simulink model "test_mdl_NI"  (R2018a)
settings: Solver=VariableStepAuto  StartTime=0.0  StopTime=10.0  RelTol=1e-3
(part 17 of 24)

== system test_mdl_NI/CAN_Signal/ECM_DIESEL PCM PCM_HEV/EngineData_7_0x179/FuelFlw_Vl_Dsply ==
  in : Inport
  out : Outport
  wires:
  in/1 -> out/1

== system test_mdl_NI/CAN_Signal/ECM_DIESEL PCM PCM_HEV/EngineData_7_0x179/HvacAirFullOut_B_Rq ==
  in : Inport
  out : Outport
  wires:
  in/1 -> out/1

== system test_mdl_NI/CAN_Signal/ECM_DIESEL PCM PCM_HEV/EngineData_7_0x179/OdoCount ==
  in : Inport
  out : Outport
  wires:
  in/1 -> out/1

== system test_mdl_NI/CAN_Signal/ECM_DIESEL PCM PCM_HEV/EngineData_7_0x179/TrnKickDown_B_RqDrv ==
  in : Inport
  out : Outport
  wires:
  in/1 -> out/1

== system test_mdl_NI/CAN_Signal/ECM_DIESEL PCM PCM_HEV/EngineData_7_0x179/TrnManShifGear_D_IndDrv ==
  in : Inport
  out : Outport
  wires:
  in/1 -> out/1

== system test_mdl_NI/CAN_Signal/ECM_DIESEL PCM PCM_HEV/EngineData_7_0x179/TrnManShif_D_IndDrv ==
  in : Inport
  out : Outport
  wires:
  in/1 -> out/1

== system test_mdl_NI/CAN_Signal/ECM_DIESEL PCM PCM_HEV/Engine_Clutch_Data_0x42F/CluPdlPosPcMeas_D_Qf ==
  in : Inport
  out : Outport
  wires:
  in/1 -> out/1

== system test_mdl_NI/CAN_Signal/ECM_DIESEL PCM PCM_HEV/Engine_Clutch_Data_0x42F/CluPdlPos_Pc_Meas ==
  in : Inport
  out : Outport
  wires:
  in/1 -> out/1

== system test_mdl_NI/CAN_Signal/ECM_DIESEL PCM PCM_HEV/Engine_Clutch_Data_0x42F/CluPdl_PcRate_Actl ==
  in : Inport
  out : Outport
  wires:
  in/1 -> out/1

== system test_mdl_NI/CAN_Signal/ECM_DIESEL PCM PCM_HEV/Engine_Clutch_Data_0x42F/EngAoutIdl_N_Ntrl ==
  in : Inport
  out : Outport
  wires:
  in/1 -> out/1

== system test_mdl_NI/CAN_Signal/ECM_DIESEL PCM PCM_HEV/Engine_Clutch_Data_0x42F/EngAout_N_Dsply ==
  in : Inport
  out : Outport
  wires:
  in/1 -> out/1

== system test_mdl_NI/CAN_Signal/ECM_DIESEL PCM PCM_HEV/Gear_Shift_by_Wire_3/GearSelLck_D_Rq ==
  in : Inport
  out : Outport
  wires:
  in/1 -> out/1

== system test_mdl_NI/CAN_Signal/ECM_DIESEL PCM PCM_HEV/Gear_Shift_by_Wire_3/PrkBrkActv_D_RqTrnGear ==
  in : Inport
  out : Outport
  wires:
  in/1 -> out/1

== system test_mdl_NI/CAN_Signal/ECM_DIESEL PCM PCM_HEV/Gear_Shift_by_Wire_3/TrnCmdCnt_B_Actl ==
  in : Inport
  out : Outport
  wires:
  in/1 -> out/1

== system test_mdl_NI/CAN_Signal/ECM_DIESEL PCM PCM_HEV/Gear_Shift_by_Wire_3/TrnCmdState_B_Actl ==
  in : Inport
  out : Outport
  wires:
  in/1 -> out/1

== system test_mdl_NI/CAN_Signal/ECM_DIESEL PCM PCM_HEV/Gear_Shift_by_Wire_3/TrnDtpCmd_D_Actl ==
  in : Inport
  out : Outport
  wires:
  in/1 -> out/1

== system test_mdl_NI/CAN_Signal/ECM_DIESEL PCM PCM_HEV/Gear_Shift_by_Wire_3/TrnGearCmd_No_Cnt ==
  in : Inport
  out : Outport
  wires:
  in/1 -> out/1

== system test_mdl_NI/CAN_Signal/ECM_DIESEL PCM PCM_HEV/Gear_Shift_by_Wire_3/TrnGearCmd_No_Cs ==
  in : Inport
  out : Outport
  wires:
  in/1 -> out/1

== system test_mdl_NI/CAN_Signal/ECM_DIESEL PCM PCM_HEV/Gear_Shift_by_Wire_3/TrnGearCmd_Pc_ActlPt ==
  in : Inport
  out : Outport
  wires:
  in/1 -> out/1

== system test_mdl_NI/CAN_Signal/ECM_DIESEL PCM PCM_HEV/Gear_Shift_by_Wire_3/TrnGearMsgTxt_D_Rq ==
  in : Inport
  out : Outport
  wires:
  in/1 -> out/1

== system test_mdl_NI/CAN_Signal/ECM_DIESEL PCM PCM_HEV/Gear_Shift_by_Wire_3/TrnGearNtmAllow_B_Stat ==
  in : Inport
  out : Outport
  wires:
  in/1 -> out/1

== system test_mdl_NI/CAN_Signal/ECM_DIESEL PCM PCM_HEV/Gear_Shift_by_Wire_3/TrnGear_D_RqPt ==
  in : Inport
  out : Outport
  wires:
  in/1 -> out/1

== system test_mdl_NI/CAN_Signal/ECM_DIESEL PCM PCM_HEV/Gear_Shift_by_Wire_3/TrnLvrV_D_Rq ==
  in : Inport
  out : Outport
  wires:
  in/1 -> out/1

== system test_mdl_NI/CAN_Signal/ECM_DIESEL PCM PCM_HEV/Gear_Shift_by_Wire_3/TrnNtrlTowCmd_D_Actl ==
  in : Inport
  out : Outport
  wires:
  in/1 -> out/1

== system test_mdl_NI/CAN_Signal/ECM_DIESEL PCM PCM_HEV/Gear_Shift_by_Wire_3/TrnSbwSysHlth_D_Actl ==
  in : Inport
  out : Outport
  wires:
  in/1 -> out/1

== system test_mdl_NI/CAN_Signal/ECM_DIESEL PCM PCM_HEV/Gear_Shift_by_Wire_3/TrnValidGear_D_Cnfm ==
  in : Inport
  out : Outport
  wires:
  in/1 -> out/1

== system test_mdl_NI/CAN_Signal/ECM_DIESEL PCM PCM_HEV/Global_PATS_TargetInfo_0x47/immoTarget1Cmd ==
  in : Inport
  out : Outport
  wires:
  in/1 -> out/1

== system test_mdl_NI/CAN_Signal/ECM_DIESEL PCM PCM_HEV/Global_PATS_TargetInfo_0x47/immoTarget1Data ==
  in : Inport
  out : Outport
  wires:
  in/1 -> out/1

== system test_mdl_NI/CAN_Signal/ECM_DIESEL PCM PCM_HEV/Global_PATS_TargetInfo_0x47/immoTarget1Status ==
  in : Inport
  out : Outport
  wires:
  in/1 -> out/1

== system test_mdl_NI/CAN_Signal/ECM_DIESEL PCM PCM_HEV/HEV_Powertrain_Data2/BattTracCnnct_D_Rq ==
  in : Inport
  out : Outport
  wires:
  in/1 -> out/1

== system test_mdl_NI/CAN_Signal/ECM_DIESEL PCM PCM_HEV/HEV_Powertrain_Data2/PrplTqMnRgen_B_Actl ==
  in : Inport
  out : Outport
  wires:
  in/1 -> out/1

== system test_mdl_NI/CAN_Signal/ECM_DIESEL PCM PCM_HEV/HEV_Powertrain_Data2/WhlDirAvgDrv_D_Actl ==
  in : Inport
  out : Outport
  wires:
  in/1 -> out/1

== system test_mdl_NI/CAN_Signal/ECM_DIESEL PCM PCM_HEV/PCM_AutoSar_NetworkMgmt_0x595/PCM_AutoSarNMControl ==
  in : Inport
  out : Outport
  wires:
  in/1 -> out/1

== system test_mdl_NI/CAN_Signal/ECM_DIESEL PCM PCM_HEV/PCM_AutoSar_NetworkMgmt_0x595/PCM_AutoSarNMNodeId ==
  in : Inport
  out : Outport
  wires:
  in/1 -> out/1

== system test_mdl_NI/CAN_Signal/ECM_DIESEL PCM PCM_HEV/PCM_AutoSar_NetworkMgmt_0x595/PCM_AutoSarNMReserved1 ==
  in : Inport
  out : Outport
  wires:
  in/1 -> out/1

== system test_mdl_NI/CAN_Signal/ECM_DIESEL PCM PCM_HEV/PCM_AutoSar_NetworkMgmt_0x595/PCM_AutoSarNMReserved2 ==
  in : Inport
  out : Outport
  wires:
  in/1 -> out/1

== system test_mdl_NI/CAN_Signal/ECM_DIESEL PCM PCM_HEV/PCM_AutoSar_NetworkMgmt_0x595/PCM_AutoSarNMReserved3 ==
  in : Inport
  out : Outport
  wires:
  in/1 -> out/1

== system test_mdl_NI/CAN_Signal/ECM_DIESEL PCM PCM_HEV/PCM_AutoSar_NetworkMgmt_0x595/PCM_AutoSarNMReserved4 ==
  in : Inport
  out : Outport
  wires:
  in/1 -> out/1

== system test_mdl_NI/CAN_Signal/ECM_DIESEL PCM PCM_HEV/PCM_AutoSar_NetworkMgmt_0x595/PCM_GWNMProxy ==
  in : Inport
  out : Outport
  wires:
  in/1 -> out/1

== system test_mdl_NI/CAN_Signal/ECM_DIESEL PCM PCM_HEV/PCM_AutoSar_NetworkMgmt_0x595/PCM_GWOnBoardTester ==
  in : Inport
  out : Outport
  wires:
  in/1 -> out/1

== system test_mdl_NI/CAN_Signal/ECM_DIESEL PCM PCM_HEV/PCM_Rapid_Data_Response_1_0x6A0/UUDTPCMResponse1 ==
  in : Inport
  out : Outport
  wires:
  in/1 -> out/1

== system test_mdl_NI/CAN_Signal/ECM_DIESEL PCM PCM_HEV/PowertrainData_10/GearEngag_D_Actl ==
  in : Inport
  out : Outport
  wires:
  in/1 -> out/1

== system test_mdl_NI/CAN_Signal/ECM_DIESEL PCM PCM_HEV/PowertrainData_10/GearLvr_D_ActlDrv ==
  in : Inport
  out : Outport
  wires:
  in/1 -> out/1

== system test_mdl_NI/CAN_Signal/ECM_DIESEL PCM PCM_HEV/PowertrainData_10/GearPos_D_Actl ==
  in : Inport
  out : Outport
  wires:
  in/1 -> out/1

== system test_mdl_NI/CAN_Signal/ECM_DIESEL PCM PCM_HEV/PowertrainData_10/GearPos_D_Trg ==
  in : Inport
  out : Outport
  wires:
  in/1 -> out/1

== system test_mdl_NI/CAN_Signal/ECM_DIESEL PCM PCM_HEV/PowertrainData_10/GearPos_No_Cnt ==
  in : Inport
  out : Outport
  wires:
  in/1 -> out/1

== system test_mdl_NI/CAN_Signal/ECM_DIESEL PCM PCM_HEV/PowertrainData_10/GearPos_No_Cs ==
  in : Inport
  out : Outport
  wires:
  in/1 -> out/1

== system test_mdl_NI/CAN_Signal/ECM_DIESEL PCM PCM_HEV/PowertrainData_10/TrnIgnOffDly_T_Rq ==
  in : Inport
  out : Outport
  wires:
  in/1 -> out/1

== system test_mdl_NI/CAN_Signal/ECM_DIESEL PCM PCM_HEV/PowertrainData_10/TrnPrkSys_D_Actl ==
  in : Inport
  out : Outport
  wires:
  in/1 -> out/1

== system test_mdl_NI/CAN_Signal/ECM_DIESEL PCM PCM_HEV/PowertrainData_10/TrnRng_D_Rq ==
  in : Inport
  out : Outport
  wires:
  in/1 -> out/1

== system test_mdl_NI/CAN_Signal/ECM_DIESEL PCM PCM_HEV/PowertrainData_1_0x421/AirCondFluidHi_P_Actl ==
  in : Inport
  out : Outport
  wires:
  in/1 -> out/1

== system test_mdl_NI/CAN_Signal/ECM_DIESEL PCM PCM_HEV/PowertrainData_1_0x421/CoolantFanStepAct ==
  in : Inport
  out : Outport
  wires:
  in/1 -> out/1

== system test_mdl_NI/CAN_Signal/ECM_DIESEL PCM PCM_HEV/PowertrainData_1_0x421/ECMMILRequest ==
  in : Inport
  out : Outport
  wires:
  in/1 -> out/1

== system test_mdl_NI/CAN_Signal/ECM_DIESEL PCM PCM_HEV/PowertrainData_1_0x421/EngIdlShutDown_D_Stat ==
  in : Inport
  out : Outport
  wires:
  in/1 -> out/1

== system test_mdl_NI/CAN_Signal/ECM_DIESEL PCM PCM_HEV/PowertrainData_1_0x421/EngIdlShutDwnTxt_D_Rq ==
  in : Inport
  out : Outport
  wires:
  in/1 -> out/1

== system test_mdl_NI/CAN_Signal/ECM_DIESEL PCM PCM_HEV/PowertrainData_1_0x421/FUEL_ALCOHOL_PERCNT ==
  in : Inport
  out : Outport
  wires:
  in/1 -> out/1

== system test_mdl_NI/CAN_Signal/ECM_DIESEL PCM PCM_HEV/PowertrainData_1_0x421/FohEng_D_Rq ==
  in : Inport
  out : Outport
  wires:
  in/1 -> out/1

== system test_mdl_NI/CAN_Signal/ECM_DIESEL PCM PCM_HEV/PowertrainData_1_0x421/OilPressureWarning ==
  in : Inport
  out : Outport
  wires:
  in/1 -> out/1

== system test_mdl_NI/CAN_Signal/ECM_DIESEL PCM PCM_HEV/PowertrainData_1_0x421/TrnTotLss_Tq_Est ==
  in : Inport
  out : Outport
  wires:
  in/1 -> out/1

== system test_mdl_NI/CAN_Signal/ECM_DIESEL PCM PCM_HEV/PowertrainData_1_0x421/TrnTotTq_Rt_Est ==
  in : Inport
  out : Outport
  wires:
  in/1 -> out/1

== system test_mdl_NI/CAN_Signal/ECM_DIESEL PCM PCM_HEV/PowertrainData_1_0x421/VehVLimActv_B_Actl ==
  in : Inport
  out : Outport
  wires:
  in/1 -> out/1

== system test_mdl_NI/CAN_Signal/ECM_DIESEL PCM PCM_HEV/PowertrainData_1_0x421/VehVLimStat_D_Actl ==
  in : Inport
  out : Outport
  wires:
  in/1 -> out/1

== system test_mdl_NI/CAN_Signal/ECM_DIESEL PCM PCM_HEV/PowertrainData_2_0x42D/ApedPos_Pc_ActlDiag ==
  in : Inport
  out : Outport
  wires:
  in/1 -> out/1

== system test_mdl_NI/CAN_Signal/ECM_DIESEL PCM PCM_HEV/PowertrainData_2_0x42D/EngAirIn_Te_Actl ==
  in : Inport
  out : Outport
  wires:
  in/1 -> out/1

== system test_mdl_NI/CAN_Signal/ECM_DIESEL PCM PCM_HEV/PowertrainData_2_0x42D/EngClnt_Te_ActlDiag ==
  in : Inport
  out : Outport
  wires:
  in/1 -> out/1

== system test_mdl_NI/CAN_Signal/ECM_DIESEL PCM PCM_HEV/PowertrainData_2_0x42D/EngLoad_Pc_CalcDiag ==
  in : Inport
  out : Outport
  wires:
  in/1 -> out/1

== system test_mdl_NI/CAN_Signal/ECM_DIESEL PCM PCM_HEV/PowertrainData_2_0x42D/EngMsgTxt_D_Rq ==
  in : Inport
  out : Outport
  wires:
  in/1 -> out/1

== system test_mdl_NI/CAN_Signal/ECM_DIESEL PCM PCM_HEV/PowertrainData_2_0x42D/GrllShtrPos_B_Falt ==
  in : Inport
  out : Outport
  wires:
  in/1 -> out/1

== system test_mdl_NI/CAN_Signal/ECM_DIESEL PCM PCM_HEV/PowertrainData_2_0x42D/GrllShtrPos_D_Cmd ==
  in : Inport
  out : Outport
  wires:
  in/1 -> out/1

== system test_mdl_NI/CAN_Signal/ECM_DIESEL PCM PCM_HEV/PowertrainData_2_0x42D/IsaOffst_D_Stat ==
  in : Inport
  out : Outport
  wires:
  in/1 -> out/1

== system test_mdl_NI/CAN_Signal/ECM_DIESEL PCM PCM_HEV/PowertrainData_2_0x42D/ObdWarmUp_B_Complt ==
  in : Inport
  out : Outport
  wires:
  in/1 -> out/1

== system test_mdl_NI/CAN_Signal/ECM_DIESEL PCM PCM_HEV/PowertrainData_2_0x42D/SlMde_D_RqDsply ==
  in : Inport
  out : Outport
  wires:
  in/1 -> out/1

== system test_mdl_NI/CAN_Signal/ECM_DIESEL PCM PCM_HEV/PowertrainData_2_0x42D/SlMde_D_Stat ==
  in : Inport
  out : Outport
  wires:
  in/1 -> out/1

== system test_mdl_NI/CAN_Signal/ECM_DIESEL PCM PCM_HEV/PowertrainData_3_0x43E/BattULoChrg_U_Cmd ==
  in : Inport
  out : Outport
  wires:
  in/1 -> out/1

== system test_mdl_NI/CAN_Signal/ECM_DIESEL PCM PCM_HEV/PowertrainData_3_0x43E/ElLoadCtl_D_Rq ==
  in : Inport
  out : Outport
  wires:
  in/1 -> out/1

== system test_mdl_NI/CAN_Signal/ECM_DIESEL PCM PCM_HEV/PowertrainData_3_0x43E/EngMnfld_P_Actl ==
  in : Inport
  out : Outport
  wires:
  in/1 -> out/1

== system test_mdl_NI/CAN_Signal/ECM_DIESEL PCM PCM_HEV/PowertrainData_3_0x43E/FuelPumpPwr_B_Rq ==
  in : Inport
  out : Outport
  wires:
  in/1 -> out/1

== system test_mdl_NI/CAN_Signal/ECM_DIESEL PCM PCM_HEV/PowertrainData_6_0x205/BrkTot_Tq_RqFapLc ==
  in : Inport
  out : Outport
  wires:
  in/1 -> out/1

== system test_mdl_NI/CAN_Signal/ECM_DIESEL PCM PCM_HEV/PowertrainData_6_0x205/FapLc_B_Err ==
  in : Inport
  out : Outport
  wires:
  in/1 -> out/1

== system test_mdl_NI/CAN_Signal/ECM_DIESEL PCM PCM_HEV/PowertrainData_6_0x205/TrnAin_Pc_RqDrv ==
  in : Inport
  out : Outport
  wires:
  in/1 -> out/1

== system test_mdl_NI/CAN_Signal/ECM_DIESEL PCM PCM_HEV/PowertrainData_7_0x41F/EcoCochA_Pc_Dsply ==
  in : Inport
  out : Outport
  wires:
  in/1 -> out/1

== system test_mdl_NI/CAN_Signal/ECM_DIESEL PCM PCM_HEV/PowertrainData_7_0x41F/EcoCochCrus_Pc_Dsply ==
  in : Inport
  out : Outport
  wires:
  in/1 -> out/1

== system test_mdl_NI/CAN_Signal/ECM_DIESEL PCM PCM_HEV/PowertrainData_7_0x41F/EcoCochDecel_Pc_Dsply ==
  in : Inport
  out : Outport
  wires:
  in/1 -> out/1

== system test_mdl_NI/CAN_Signal/ECM_DIESEL PCM PCM_HEV/PowertrainData_7_0x41F/EcoCochIdlFuel_Pc_Dsply ==
  in : Inport
  out : Outport
  wires:
  in/1 -> out/1

== system test_mdl_NI/CAN_Signal/ECM_DIESEL PCM PCM_HEV/PowertrainData_7_0x41F/EcoCochInstNeg_B_Dsply ==
  in : Inport
  out : Outport
  wires:
  in/1 -> out/1

== system test_mdl_NI/CAN_Signal/ECM_DIESEL PCM PCM_HEV/PowertrainData_7_0x41F/EcoCochInst_Pc_Dsply ==
  in : Inport
  out : Outport
  wires:
  in/1 -> out/1

== system test_mdl_NI/CAN_Signal/ECM_DIESEL PCM PCM_HEV/PowertrainData_7_0x41F/EcoCochShif_Pc_Dsply ==
  in : Inport
  out : Outport
  wires:
  in/1 -> out/1

== system test_mdl_NI/CAN_Signal/ECM_DIESEL PCM PCM_HEV/PowertrainData_9_0x44C/AutoTowActv_B_Stat ==
  in : Inport
  out : Outport
  wires:
  in/1 -> out/1

== system test_mdl_NI/CAN_Signal/ECM_DIESEL PCM PCM_HEV/PowertrainData_9_0x44C/AutoTowAllw_D_StatMnu ==
  in : Inport
  out : Outport
  wires:
  in/1 -> out/1

== system test_mdl_NI/CAN_Signal/ECM_DIESEL PCM PCM_HEV/PowertrainData_9_0x44C/GrossTrainWeight_M_Est ==
  in : Inport
  out : Outport
  wires:
  in/1 -> out/1

== system test_mdl_NI/CAN_Signal/ECM_DIESEL PCM PCM_HEV/PowertrainData_9_0x44C/TrailCtlPt_B_Falt ==
  in : Inport
  out : Outport
  wires:
  in/1 -> out/1

== system test_mdl_NI/CAN_Signal/ECM_DIESEL PCM PCM_HEV/PowertrainData_9_0x44C/Veh_V_DsplyTrailCtlSet ==
  in : Inport
  out : Outport
  wires:
  in/1 -> out/1

== system test_mdl_NI/CAN_Signal/ECM_DIESEL PCM PCM_HEV/PowertrainData_9_0x44C/WakeAlarm1_B_Typ ==
  in : Inport
  out : Outport
  wires:
  in/1 -> out/1

== system test_mdl_NI/CAN_Signal/ECM_DIESEL PCM PCM_HEV/PowertrainData_9_0x44C/WakeAlarm1_T_Rq ==
  in : Inport
  out : Outport
  wires:
  in/1 -> out/1

== system test_mdl_NI/CAN_Signal/ECM_DIESEL PCM PCM_HEV/Powertrain_Data_4_0x424/BpedDrvMsgTxt_B_Dsply ==
  in : Inport
  out : Outport
  wires:
  in/1 -> out/1

== system test_mdl_NI/CAN_Signal/ECM_DIESEL PCM PCM_HEV/Powertrain_Data_4_0x424/FuelLvlWarn_D_ActlEng ==
  in : Inport
  out : Outport
  wires:
  in/1 -> out/1

== system test_mdl_NI/CAN_Signal/ECM_DIESEL PCM PCM_HEV/Powertrain_Data_4_0x424/FuelLvl_Pc_DsplyEng ==
  in : Inport
  out : Outport
  wires:
  in/1 -> out/1

== system test_mdl_NI/CAN_Signal/ECM_DIESEL PCM PCM_HEV/Powertrain_Data_4_0x424/FuelRange_L_DsplyEng ==
  in : Inport
  out : Outport
  wires:
  in/1 -> out/1

== system test_mdl_NI/CAN_Signal/ECM_DIESEL PCM PCM_HEV/Powertrain_Data_4_0x424/RearDiffOilTeWarn_B_Rq ==
  in : Inport
  out : Outport
  wires:
  in/1 -> out/1

== system test_mdl_NI/CAN_Signal/ECM_DIESEL PCM PCM_HEV/Powertrain_Data_4_0x424/RearDiffOil_Te_Actl ==
  in : Inport
  out : Outport
  wires:
  in/1 -> out/1

== system test_mdl_NI/CAN_Signal/ECM_DIESEL PCM PCM_HEV/Powertrain_Data_4_0x424/SelDrvMdePt_D_Stat ==
  in : Inport
  out : Outport
  wires:
  in/1 -> out/1

== system test_mdl_NI/CAN_Signal/ECM_DIESEL PCM PCM_HEV/Powertrain_Data_5_0x43F/FapLcActv_B_Stat ==
  in : Inport
  out : Outport
  wires:
  in/1 -> out/1

== system test_mdl_NI/CAN_Signal/ECM_DIESEL PCM PCM_HEV/Powertrain_Data_5_0x43F/FapLcInhbt_B_Rq ==
  in : Inport
  out : Outport
  wires:
  in/1 -> out/1

== system test_mdl_NI/CAN_Signal/ECM_DIESEL PCM PCM_HEV/Powertrain_Data_5_0x43F/FapLcMaxGrdAbrt_B_Stat ==
  in : Inport
  out : Outport
  wires:
  in/1 -> out/1

== system test_mdl_NI/CAN_Signal/ECM_DIESEL PCM PCM_HEV/Powertrain_Data_5_0x43F/FapLcMaxGrdInhbt_B_Stat ==
  in : Inport
  out : Outport
  wires:
  in/1 -> out/1

== system test_mdl_NI/CAN_Signal/ECM_DIESEL PCM PCM_HEV/Powertrain_Data_5_0x43F/FapLcObstcl_B_Stat ==
  in : Inport
  out : Outport
  wires:
  in/1 -> out/1

== system test_mdl_NI/CAN_Signal/ECM_DIESEL PCM PCM_HEV/Powertrain_Data_5_0x43F/FapLcPrchgBrk_B_Rq ==
  in : Inport
  out : Outport
  wires:
  in/1 -> out/1

== system test_mdl_NI/CAN_Signal/ECM_DIESEL PCM PCM_HEV/Powertrain_Data_5_0x43F/FapLcStopHold_B_Rq ==
  in : Inport
  out : Outport
  wires:
  in/1 -> out/1

== system test_mdl_NI/CAN_Signal/ECM_DIESEL PCM PCM_HEV/Stop_Start_0x166/AutoStopPtDelta_I_Est ==
  in : Inport
  out : Outport
  wires:
  in/1 -> out/1

== system test_mdl_NI/CAN_Signal/ECM_DIESEL PCM PCM_HEV/Stop_Start_0x166/HiElPwInhbt_B_Stat ==
  in : Inport
  out : Outport
  wires:
  in/1 -> out/1

== system test_mdl_NI/CAN_Signal/ECM_DIESEL PCM PCM_HEV/Stop_Start_0x166/OdoTripVerify_L_Actl ==
  in : Inport
  out : Outport
  wires:
  in/1 -> out/1

== system test_mdl_NI/CAN_Signal/ECM_DIESEL PCM PCM_HEV/Stop_Start_0x166/StopStrtDrvMde_D_Indic ==
  in : Inport
  out : Outport
  wires:
  in/1 -> out/1

== system test_mdl_NI/CAN_Signal/ECM_DIESEL PCM PCM_HEV/Stop_Start_0x166/StopStrtIODTxt_D_Rq ==
  in : Inport
  out : Outport
  wires:
  in/1 -> out/1

== system test_mdl_NI/CAN_Signal/ECM_DIESEL PCM PCM_HEV/Stop_Start_0x166/StopStrtMsgTxt_D_Rq ==
  in : Inport
  out : Outport
  wires:
  in/1 -> out/1

== system test_mdl_NI/CAN_Signal/ECM_DIESEL PCM PCM_HEV/Stop_Start_0x166/StopStrtStdby_D_Indic ==
  in : Inport
  out : Outport
  wires:
  in/1 -> out/1

== system test_mdl_NI/CAN_Signal/ECM_DIESEL PCM PCM_HEV/TesterPhysicalResPCM_0x7E8/TesterPhysicalResPCM ==
  in : Inport
  out : Outport
  wires:
  in/1 -> out/1

== system test_mdl_NI/CAN_Signal/ECM_DIESEL PCM PCM_HEV/TorqueDataEngFlags_0x200/PrplWhlTotTqRq_No_Cnt ==
  in : Inport
  out : Outport
  wires:
  in/1 -> out/1

== system test_mdl_NI/CAN_Signal/ECM_DIESEL PCM PCM_HEV/TorqueDataEngFlags_0x200/PrplWhlTotTqRq_No_Cs ==
  in : Inport
  out : Outport
  wires:
  in/1 -> out/1

== system test_mdl_NI/CAN_Signal/ECM_DIESEL PCM PCM_HEV/TorqueDataEngFlags_0x200/PrplWhlTot_Tq_LimMn ==
  in : Inport
  out : Outport
  wires:
  in/1 -> out/1

== system test_mdl_NI/CAN_Signal/ECM_DIESEL PCM PCM_HEV/TorqueDataEngFlags_0x200/PrplWhlTot_Tq_Rq ==
  in : Inport
  out : Outport
  wires:
  in/1 -> out/1

== system test_mdl_NI/CAN_Signal/ECM_DIESEL PCM PCM_HEV/TorqueDataEngFlags_0x200/PtDrvMde_D_Stat ==
  in : Inport
  out : Outport
  wires:
  in/1 -> out/1

== system test_mdl_NI/CAN_Signal/ECM_DIESEL PCM PCM_HEV/TransGearData/GboxOil_Te_Actl ==
  in : Inport
  out : Outport
  wires:
  in/1 -> out/1

== system test_mdl_NI/CAN_Signal/ECM_DIESEL PCM PCM_HEV/TransGearData/GearLvrPos_D_Actl ==
  in : Inport
  out : Outport
  wires:
  in/1 -> out/1

== system test_mdl_NI/CAN_Signal/ECM_DIESEL PCM PCM_HEV/TransGearData/SelDrvMdeSwtch_D_Stat3 ==
  in : Inport
  out : Outport
  wires:
  in/1 -> out/1

== system test_mdl_NI/CAN_Signal/ECM_DIESEL PCM PCM_HEV/TransGearData/TrnShifActv_B_Actl ==
  in : Inport
  out : Outport
  wires:
  in/1 -> out/1

== system test_mdl_NI/CAN_Signal/ECM_DIESEL PCM PCM_HEV/TransGearData/TrnSrvcRqd_B_Rq ==
  in : Inport
  out : Outport
  wires:
  in/1 -> out/1

== system test_mdl_NI/CAN_Signal/ECM_DIESEL PCM PCM_HEV/VehicleOperatingModes_0x167/ElPw_D_Stat ==
  in : Inport
  out : Outport
  wires:
  in/1 -> out/1

== system test_mdl_NI/CAN_Signal/ECM_DIESEL PCM PCM_HEV/VehicleOperatingModes_0x167/ElPw_D_StatStrtStop ==
  in : Inport
  out : Outport
  wires:
  in/1 -> out/1

== system test_mdl_NI/CAN_Signal/ECM_DIESEL PCM PCM_HEV/VehicleOperatingModes_0x167/Eng_D_Stat ==
  in : Inport
  out : Outport
  wires:
  in/1 -> out/1

== system test_mdl_NI/CAN_Signal/ECM_DIESEL PCM PCM_HEV/VehicleOperatingModes_0x167/PlgActvArb_B_Actl ==
  in : Inport
  out : Outport
  wires:
  in/1 -> out/1

== system test_mdl_NI/CAN_Signal/ECM_DIESEL PCM PCM_HEV/VehicleOperatingModes_0x167/PrplWhlRgenMn_Tq_Actl ==
  in : Inport
  out : Outport
  wires:
  in/1 -> out/1

== system test_mdl_NI/CAN_Signal/ECM_DIESEL PCM PCM_HEV/VehicleOperatingModes_0x167/PrplWhlTot2_Tq_Actl ==
  in : Inport
  out : Outport
  wires:
  in/1 -> out/1

== system test_mdl_NI/CAN_Signal/ECM_DIESEL PCM PCM_HEV/VehicleOperatingModes_0x167/PwPckTq_D_Stat ==
  in : Inport
  out : Outport
  wires:
  in/1 -> out/1

== system test_mdl_NI/CAN_Signal/ECM_DIESEL PCM PCM_HEV/VehicleOperatingModes_0x167/TrnAinTq_D_Qf ==
  in : Inport
  out : Outport
  wires:
  in/1 -> out/1

== system test_mdl_NI/CAN_Signal/ECM_DIESEL PCM PCM_HEV/VehicleOperatingModes_0x167/TrnAin_Tq_Actl ==
  in : Inport
  out : Outport
  wires:
  in/1 -> out/1

== system test_mdl_NI/CAN_Signal/GWM/GSM/Gear_Shift_by_Wire_2_FD1_168 ==
  in : Inport
  GearButtnStuck_B_Actl : Subsystem
  GsmSrvcRqd_B_Rq : Subsystem
  TrnGearPwmFalt_B_Actl : Subsystem
  TrnTrcmPwmSig_D_Actl : Subsystem
  bus_creator : BusCreator  Inputs=4
  bus_selector : BusSelector  OutputSignals=GearButtnStuck_B_Actl,GsmSrvcRqd_B_Rq,TrnGearPwmFalt_B_Actl,TrnTrcmPwmSig_D_Actl
  out_port : Outport
  wires:
  bus_creator/1 -> out_port/1  "Gear_Shift_by_Wire_2_FD1_168"
  GearButtnStuck_B_Actl/1(out) -> bus_creator/1  "GearButtnStuck_B_Actl"
  GsmSrvcRqd_B_Rq/1(out) -> bus_creator/2  "GsmSrvcRqd_B_Rq"
  TrnGearPwmFalt_B_Actl/1(out) -> bus_creator/3  "TrnGearPwmFalt_B_Actl"
  TrnTrcmPwmSig_D_Actl/1(out) -> bus_creator/4  "TrnTrcmPwmSig_D_Actl"
  bus_selector/1 -> GearButtnStuck_B_Actl/1(in)  "<GearButtnStuck_B_Actl>"
  bus_selector/2 -> GsmSrvcRqd_B_Rq/1(in)  "<GsmSrvcRqd_B_Rq>"
  bus_selector/3 -> TrnGearPwmFalt_B_Actl/1(in)  "<TrnGearPwmFalt_B_Actl>"
  bus_selector/4 -> TrnTrcmPwmSig_D_Actl/1(in)  "<TrnTrcmPwmSig_D_Actl>"
  in/1 -> bus_selector/1

== system test_mdl_NI/CAN_Signal/GWM/GSM/Gear_Shift_by_Wire_FD1_5A ==
  in : Inport
  BrkSwtchPos_B_ActlGsm : Subsystem
  DrQltyDrv_D_StatGsm : Subsystem
  GsmGearMsgTxt_D_Rq : Subsystem
  PrkBrkActv_D_RqGsmGear : Subsystem
  TrnBtsiOvrrd_B_Stat : Subsystem
  TrnGearButtn_B_ActlD0 : Subsystem
  TrnGearButtn_B_ActlD1 : Subsystem
  TrnGearButtn_B_ActlD2 : Subsystem
  TrnGearButtn_B_ActlM0 : Subsystem
  TrnGearButtn_B_ActlM1 : Subsystem
  TrnGearButtn_B_ActlM2 : Subsystem
  TrnGearButtn_B_ActlN0 : Subsystem
  TrnGearButtn_B_ActlN1 : Subsystem
  TrnGearButtn_B_ActlN2 : Subsystem
  TrnGearButtn_B_ActlP0 : Subsystem
  TrnGearButtn_B_ActlP1 : Subsystem
  TrnGearButtn_B_ActlP2 : Subsystem
  TrnGearButtn_B_ActlR0 : Subsystem
  TrnGearButtn_B_ActlR1 : Subsystem
  TrnGearButtn_B_ActlR2 : Subsystem
  TrnGearButtn_U_Actl : Subsystem
  TrnGearRqCnt_B_Actl : Subsystem
  TrnGear_D_RqDrv : Subsystem
  TrnGear_No_Cnt : Subsystem
  TrnGear_No_Cs : Subsystem
  TrnGsmNtmState_D_Actl : Subsystem
  TrnRng_D_RqGsm : Subsystem
  TrnValidGearRq_D_Stat : Subsystem
  bus_creator : BusCreator  Inputs=28
  bus_selector : BusSelector  OutputSignals=BrkSwtchPos_B_ActlGsm,DrQltyDrv_D_StatGsm,GsmGearMsgTxt_D_Rq,PrkBrkActv_D_RqGsmGear,TrnBtsiOvrrd_B_Stat,TrnGearButtn_B_ActlD0,TrnGearButtn_B_ActlD1,TrnGearButtn_B_ActlD2,TrnGearButtn_B_ActlM0,TrnGearButtn_B_ActlM1,TrnGearButtn_B_ActlM2,TrnGearButtn_B_ActlN0,TrnGearButtn_B_ActlN1,TrnGearButtn_B_ActlN2,TrnGearButtn_B_ActlP0,TrnGearButtn_B_ActlP1,TrnGearButtn_B_ActlP2,TrnGearButtn_B_ActlR0,TrnGearButtn_B_ActlR1,TrnGearButtn_B_ActlR2,TrnGearButtn_U_Actl,TrnGearRqCnt_B_Actl,TrnGear_D_RqDrv,TrnGear_No_Cnt,TrnGear_No_Cs,TrnGsmNtmState_D_Actl,TrnRng_D_RqGsm,TrnValidGearRq_D_Stat
  out_port : Outport
  wires:
  bus_creator/1 -> out_port/1  "Gear_Shift_by_Wire_FD1_5A"
  BrkSwtchPos_B_ActlGsm/1(out) -> bus_creator/1  "BrkSwtchPos_B_ActlGsm"
  DrQltyDrv_D_StatGsm/1(out) -> bus_creator/2  "DrQltyDrv_D_StatGsm"
  GsmGearMsgTxt_D_Rq/1(out) -> bus_creator/3  "GsmGearMsgTxt_D_Rq"
  PrkBrkActv_D_RqGsmGear/1(out) -> bus_creator/4  "PrkBrkActv_D_RqGsmGear"
  TrnBtsiOvrrd_B_Stat/1(out) -> bus_creator/5  "TrnBtsiOvrrd_B_Stat"
  TrnGearButtn_B_ActlD0/1(out) -> bus_creator/6  "TrnGearButtn_B_ActlD0"
  TrnGearButtn_B_ActlD1/1(out) -> bus_creator/7  "TrnGearButtn_B_ActlD1"
  TrnGearButtn_B_ActlD2/1(out) -> bus_creator/8  "TrnGearButtn_B_ActlD2"
  TrnGearButtn_B_ActlM0/1(out) -> bus_creator/9  "TrnGearButtn_B_ActlM0"
  TrnGearButtn_B_ActlM1/1(out) -> bus_creator/10  "TrnGearButtn_B_ActlM1"
  TrnGearButtn_B_ActlM2/1(out) -> bus_creator/11  "TrnGearButtn_B_ActlM2"
  TrnGearButtn_B_ActlN0/1(out) -> bus_creator/12  "TrnGearButtn_B_ActlN0"
  TrnGearButtn_B_ActlN1/1(out) -> bus_creator/13  "TrnGearButtn_B_ActlN1"
  TrnGearButtn_B_ActlN2/1(out) -> bus_creator/14  "TrnGearButtn_B_ActlN2"
  TrnGearButtn_B_ActlP0/1(out) -> bus_creator/15  "TrnGearButtn_B_ActlP0"
  TrnGearButtn_B_ActlP1/1(out) -> bus_creator/16  "TrnGearButtn_B_ActlP1"
  TrnGearButtn_B_ActlP2/1(out) -> bus_creator/17  "TrnGearButtn_B_ActlP2"
  TrnGearButtn_B_ActlR0/1(out) -> bus_creator/18  "TrnGearButtn_B_ActlR0"
  TrnGearButtn_B_ActlR1/1(out) -> bus_creator/19  "TrnGearButtn_B_ActlR1"
  TrnGearButtn_B_ActlR2/1(out) -> bus_creator/20  "TrnGearButtn_B_ActlR2"
  TrnGearButtn_U_Actl/1(out) -> bus_creator/21  "TrnGearButtn_U_Actl"
  TrnGearRqCnt_B_Actl/1(out) -> bus_creator/22  "TrnGearRqCnt_B_Actl"
  TrnGear_D_RqDrv/1(out) -> bus_creator/23  "TrnGear_D_RqDrv"
  TrnGear_No_Cnt/1(out) -> bus_creator/24  "TrnGear_No_Cnt"
  TrnGear_No_Cs/1(out) -> bus_creator/25  "TrnGear_No_Cs"
  TrnGsmNtmState_D_Actl/1(out) -> bus_creator/26  "TrnGsmNtmState_D_Actl"
  TrnRng_D_RqGsm/1(out) -> bus_creator/27  "TrnRng_D_RqGsm"
  TrnValidGearRq_D_Stat/1(out) -> bus_creator/28  "TrnValidGearRq_D_Stat"
  bus_selector/1 -> BrkSwtchPos_B_ActlGsm/1(in)  "<BrkSwtchPos_B_ActlGsm>"
  bus_selector/2 -> DrQltyDrv_D_StatGsm/1(in)  "<DrQltyDrv_D_StatGsm>"
  bus_selector/3 -> GsmGearMsgTxt_D_Rq/1(in)  "<GsmGearMsgTxt_D_Rq>"
  bus_selector/4 -> PrkBrkActv_D_RqGsmGear/1(in)  "<PrkBrkActv_D_RqGsmGear>"
  bus_selector/5 -> TrnBtsiOvrrd_B_Stat/1(in)  "<TrnBtsiOvrrd_B_Stat>"
  bus_selector/6 -> TrnGearButtn_B_ActlD0/1(in)  "<TrnGearButtn_B_ActlD0>"
  bus_selector/7 -> TrnGearButtn_B_ActlD1/1(in)  "<TrnGearButtn_B_ActlD1>"
  bus_selector/8 -> TrnGearButtn_B_ActlD2/1(in)  "<TrnGearButtn_B_ActlD2>"
  bus_selector/9 -> TrnGearButtn_B_ActlM0/1(in)  "<TrnGearButtn_B_ActlM0>"
  bus_selector/10 -> TrnGearButtn_B_ActlM1/1(in)  "<TrnGearButtn_B_ActlM1>"
  bus_selector/11 -> TrnGearButtn_B_ActlM2/1(in)  "<TrnGearButtn_B_ActlM2>"
  bus_selector/12 -> TrnGearButtn_B_ActlN0/1(in)  "<TrnGearButtn_B_ActlN0>"
  bus_selector/13 -> TrnGearButtn_B_ActlN1/1(in)  "<TrnGearButtn_B_ActlN1>"
  bus_selector/14 -> TrnGearButtn_B_ActlN2/1(in)  "<TrnGearButtn_B_ActlN2>"
  bus_selector/15 -> TrnGearButtn_B_ActlP0/1(in)  "<TrnGearButtn_B_ActlP0>"
  bus_selector/16 -> TrnGearButtn_B_ActlP1/1(in)  "<TrnGearButtn_B_ActlP1>"
  bus_selector/17 -> TrnGearButtn_B_ActlP2/1(in)  "<TrnGearButtn_B_ActlP2>"
  bus_selector/18 -> TrnGearButtn_B_ActlR0/1(in)  "<TrnGearButtn_B_ActlR0>"
  bus_selector/19 -> TrnGearButtn_B_ActlR1/1(in)  "<TrnGearButtn_B_ActlR1>"
  bus_selector/20 -> TrnGearButtn_B_ActlR2/1(in)  "<TrnGearButtn_B_ActlR2>"
  bus_selector/21 -> TrnGearButtn_U_Actl/1(in)  "<TrnGearButtn_U_Actl>"
  bus_selector/22 -> TrnGearRqCnt_B_Actl/1(in)  "<TrnGearRqCnt_B_Actl>"
  bus_selector/23 -> TrnGear_D_RqDrv/1(in)  "<TrnGear_D_RqDrv>"
  bus_selector/24 -> TrnGear_No_Cnt/1(in)  "<TrnGear_No_Cnt>"
  bus_selector/25 -> TrnGear_No_Cs/1(in)  "<TrnGear_No_Cs>"
  bus_selector/26 -> TrnGsmNtmState_D_Actl/1(in)  "<TrnGsmNtmState_D_Actl>"
  bus_selector/27 -> TrnRng_D_RqGsm/1(in)  "<TrnRng_D_RqGsm>"
  bus_selector/28 -> TrnValidGearRq_D_Stat/1(in)  "<TrnValidGearRq_D_Stat>"
  in/1 -> bus_selector/1

== system test_mdl_NI/CAN_Signal/GWM/Other_GWMTx/AC_Compressor_Data_FD1 ==
  in : Inport
  ElCmprBattSysU_D_Falt : Subsystem
  ElCmprBattURng_D_Falt : Subsystem
  ElCmprInnrErr_D_Falt : Subsystem
  ElCmprLostComm_D_Falt : Subsystem
  ElCmprOverLoad_D_Falt : Subsystem
  ElCmprOverTe_D_Falt : Subsystem
  ElCmprOverTe_D_Stat : Subsystem
  ElCmprPerfErr_D_Falt : Subsystem
  ElCmprSysU_D_Falt : Subsystem
  ElCmprUHi_D_Stat : Subsystem
  ElCmprUHi_U_Actl : Subsystem
  ElCmpr_D_Stat : Subsystem
  ElCmpr_N_Actl : Subsystem
  ElCmpr_Pw_Actl : Subsystem
  bus_creator : BusCreator  Inputs=14
  bus_selector : BusSelector  OutputSignals=ElCmprBattSysU_D_Falt,ElCmprBattURng_D_Falt,ElCmprInnrErr_D_Falt,ElCmprLostComm_D_Falt,ElCmprOverLoad_D_Falt,ElCmprOverTe_D_Falt,ElCmprOverTe_D_Stat,ElCmprPerfErr_D_Falt,ElCmprSysU_D_Falt,ElCmprUHi_D_Stat,ElCmprUHi_U_Actl,ElCmpr_D_Stat,ElCmpr_N_Actl,ElCmpr_Pw_Actl
  out_port : Outport
  wires:
  bus_creator/1 -> out_port/1  "AC_Compressor_Data_FD1"
  ElCmprBattSysU_D_Falt/1(out) -> bus_creator/1  "ElCmprBattSysU_D_Falt"
  ElCmprBattURng_D_Falt/1(out) -> bus_creator/2  "ElCmprBattURng_D_Falt"
  ElCmprInnrErr_D_Falt/1(out) -> bus_creator/3  "ElCmprInnrErr_D_Falt"
  ElCmprLostComm_D_Falt/1(out) -> bus_creator/4  "ElCmprLostComm_D_Falt"
  ElCmprOverLoad_D_Falt/1(out) -> bus_creator/5  "ElCmprOverLoad_D_Falt"
  ElCmprOverTe_D_Falt/1(out) -> bus_creator/6  "ElCmprOverTe_D_Falt"
  ElCmprOverTe_D_Stat/1(out) -> bus_creator/7  "ElCmprOverTe_D_Stat"
  ElCmprPerfErr_D_Falt/1(out) -> bus_creator/8  "ElCmprPerfErr_D_Falt"
  ElCmprSysU_D_Falt/1(out) -> bus_creator/9  "ElCmprSysU_D_Falt"
  ElCmprUHi_D_Stat/1(out) -> bus_creator/10  "ElCmprUHi_D_Stat"
  ElCmprUHi_U_Actl/1(out) -> bus_creator/11  "ElCmprUHi_U_Actl"
  ElCmpr_D_Stat/1(out) -> bus_creator/12  "ElCmpr_D_Stat"
  ElCmpr_N_Actl/1(out) -> bus_creator/13  "ElCmpr_N_Actl"
  ElCmpr_Pw_Actl/1(out) -> bus_creator/14  "ElCmpr_Pw_Actl"
  bus_selector/1 -> ElCmprBattSysU_D_Falt/1(in)  "<ElCmprBattSysU_D_Falt>"
  bus_selector/2 -> ElCmprBattURng_D_Falt/1(in)  "<ElCmprBattURng_D_Falt>"
  bus_selector/3 -> ElCmprInnrErr_D_Falt/1(in)  "<ElCmprInnrErr_D_Falt>"
  bus_selector/4 -> ElCmprLostComm_D_Falt/1(in)  "<ElCmprLostComm_D_Falt>"
  bus_selector/5 -> ElCmprOverLoad_D_Falt/1(in)  "<ElCmprOverLoad_D_Falt>"
  bus_selector/6 -> ElCmprOverTe_D_Falt/1(in)  "<ElCmprOverTe_D_Falt>"
  bus_selector/7 -> ElCmprOverTe_D_Stat/1(in)  "<ElCmprOverTe_D_Stat>"
  bus_selector/8 -> ElCmprPerfErr_D_Falt/1(in)  "<ElCmprPerfErr_D_Falt>"
  bus_selector/9 -> ElCmprSysU_D_Falt/1(in)  "<ElCmprSysU_D_Falt>"
  bus_selector/10 -> ElCmprUHi_D_Stat/1(in)  "<ElCmprUHi_D_Stat>"
  bus_selector/11 -> ElCmprUHi_U_Actl/1(in)  "<ElCmprUHi_U_Actl>"
  bus_selector/12 -> ElCmpr_D_Stat/1(in)  "<ElCmpr_D_Stat>"
  bus_selector/13 -> ElCmpr_N_Actl/1(in)  "<ElCmpr_N_Actl>"
  bus_selector/14 -> ElCmpr_Pw_Actl/1(in)  "<ElCmpr_Pw_Actl>"
  in/1 -> bus_selector/1

== system test_mdl_NI/CAN_Signal/GWM/Other_GWMTx/AC_Compressor_Req_FD1 ==
  in : Inport
  ElCmprEnbl_B_Rq : Subsystem
  ElCmpr_N_Rq : Subsystem
  bus_creator : BusCreator  Inputs=2
  bus_selector : BusSelector  OutputSignals=ElCmprEnbl_B_Rq,ElCmpr_N_Rq
  out_port : Outport
  wires:
  bus_creator/1 -> out_port/1  "AC_Compressor_Req_FD1"
  ElCmprEnbl_B_Rq/1(out) -> bus_creator/1  "ElCmprEnbl_B_Rq"
  ElCmpr_N_Rq/1(out) -> bus_creator/2  "ElCmpr_N_Rq"
  bus_selector/1 -> ElCmprEnbl_B_Rq/1(in)  "<ElCmprEnbl_B_Rq>"
  bus_selector/2 -> ElCmpr_N_Rq/1(in)  "<ElCmpr_N_Rq>"
  in/1 -> bus_selector/1

== system test_mdl_NI/CAN_Signal/GWM/Other_GWMTx/APIMGPS_Data_Nav_1_FD1 ==
  in : Inport
  GPS_Latitude_Degrees : Subsystem
  GPS_Latitude_Min_dec : Subsystem
  GPS_Latitude_Minutes : Subsystem
  GPS_Longitude_Degrees : Subsystem
  GPS_Longitude_Min_dec : Subsystem
  GPS_Longitude_Minutes : Subsystem
  GpsHsphLattSth_D_Actl : Subsystem
  GpsHsphLongEast_D_Actl : Subsystem
  bus_creator : BusCreator  Inputs=8
  bus_selector : BusSelector  OutputSignals=GPS_Latitude_Degrees,GPS_Latitude_Min_dec,GPS_Latitude_Minutes,GPS_Longitude_Degrees,GPS_Longitude_Min_dec,GPS_Longitude_Minutes,GpsHsphLattSth_D_Actl,GpsHsphLongEast_D_Actl
  out_port : Outport
  wires:
  bus_creator/1 -> out_port/1  "APIMGPS_Data_Nav_1_FD1"
  GPS_Latitude_Degrees/1(out) -> bus_creator/1  "GPS_Latitude_Degrees"
  GPS_Latitude_Min_dec/1(out) -> bus_creator/2  "GPS_Latitude_Min_dec"
  GPS_Latitude_Minutes/1(out) -> bus_creator/3  "GPS_Latitude_Minutes"
  GPS_Longitude_Degrees/1(out) -> bus_creator/4  "GPS_Longitude_Degrees"
  GPS_Longitude_Min_dec/1(out) -> bus_creator/5  "GPS_Longitude_Min_dec"
  GPS_Longitude_Minutes/1(out) -> bus_creator/6  "GPS_Longitude_Minutes"
  GpsHsphLattSth_D_Actl/1(out) -> bus_creator/7  "GpsHsphLattSth_D_Actl"
  GpsHsphLongEast_D_Actl/1(out) -> bus_creator/8  "GpsHsphLongEast_D_Actl"
  bus_selector/1 -> GPS_Latitude_Degrees/1(in)  "<GPS_Latitude_Degrees>"
  bus_selector/2 -> GPS_Latitude_Min_dec/1(in)  "<GPS_Latitude_Min_dec>"
  bus_selector/3 -> GPS_Latitude_Minutes/1(in)  "<GPS_Latitude_Minutes>"
  bus_selector/4 -> GPS_Longitude_Degrees/1(in)  "<GPS_Longitude_Degrees>"
  bus_selector/5 -> GPS_Longitude_Min_dec/1(in)  "<GPS_Longitude_Min_dec>"
  bus_selector/6 -> GPS_Longitude_Minutes/1(in)  "<GPS_Longitude_Minutes>"
  bus_selector/7 -> GpsHsphLattSth_D_Actl/1(in)  "<GpsHsphLattSth_D_Actl>"
  bus_selector/8 -> GpsHsphLongEast_D_Actl/1(in)  "<GpsHsphLongEast_D_Actl>"
  in/1 -> bus_selector/1

== system test_mdl_NI/CAN_Signal/GWM/Other_GWMTx/APIMGPS_Data_Nav_2_FD1 ==
  in : Inport
  GPS_Actual_vs_Infer_pos : Subsystem
  GPS_Compass_direction : Subsystem
  GPS_Pdop : Subsystem
  GPS_UTC_hours : Subsystem
  GPS_UTC_minutes : Subsystem
  GPS_UTC_seconds : Subsystem
  GpsUtcDay_No_Actl : Subsystem
  GpsUtcMnth_No_Actl : Subsystem
  GpsUtcYr_No_Actl : Subsystem
  Gps_B_Falt : Subsystem
  bus_creator : BusCreator  Inputs=10
  bus_selector : BusSelector  OutputSignals=GPS_Actual_vs_Infer_pos,GPS_Compass_direction,GPS_Pdop,GPS_UTC_hours,GPS_UTC_minutes,GPS_UTC_seconds,GpsUtcDay_No_Actl,GpsUtcMnth_No_Actl,GpsUtcYr_No_Actl,Gps_B_Falt
  out_port : Outport
  wires:
  bus_creator/1 -> out_port/1  "APIMGPS_Data_Nav_2_FD1"
  GPS_Actual_vs_Infer_pos/1(out) -> bus_creator/1  "GPS_Actual_vs_Infer_pos"
  GPS_Compass_direction/1(out) -> bus_creator/2  "GPS_Compass_direction"
  GPS_Pdop/1(out) -> bus_creator/3  "GPS_Pdop"
  GPS_UTC_hours/1(out) -> bus_creator/4  "GPS_UTC_hours"
  GPS_UTC_minutes/1(out) -> bus_creator/5  "GPS_UTC_minutes"
  GPS_UTC_seconds/1(out) -> bus_creator/6  "GPS_UTC_seconds"
  GpsUtcDay_No_Actl/1(out) -> bus_creator/7  "GpsUtcDay_No_Actl"
  GpsUtcMnth_No_Actl/1(out) -> bus_creator/8  "GpsUtcMnth_No_Actl"
  GpsUtcYr_No_Actl/1(out) -> bus_creator/9  "GpsUtcYr_No_Actl"
  Gps_B_Falt/1(out) -> bus_creator/10  "Gps_B_Falt"
  bus_selector/1 -> GPS_Actual_vs_Infer_pos/1(in)  "<GPS_Actual_vs_Infer_pos>"
  bus_selector/2 -> GPS_Compass_direction/1(in)  "<GPS_Compass_direction>"
  bus_selector/3 -> GPS_Pdop/1(in)  "<GPS_Pdop>"
  bus_selector/4 -> GPS_UTC_hours/1(in)  "<GPS_UTC_hours>"
  bus_selector/5 -> GPS_UTC_minutes/1(in)  "<GPS_UTC_minutes>"
  bus_selector/6 -> GPS_UTC_seconds/1(in)  "<GPS_UTC_seconds>"
  bus_selector/7 -> GpsUtcDay_No_Actl/1(in)  "<GpsUtcDay_No_Actl>"
  bus_selector/8 -> GpsUtcMnth_No_Actl/1(in)  "<GpsUtcMnth_No_Actl>"
  bus_selector/9 -> GpsUtcYr_No_Actl/1(in)  "<GpsUtcYr_No_Actl>"
  bus_selector/10 -> Gps_B_Falt/1(in)  "<Gps_B_Falt>"
  in/1 -> bus_selector/1

== system test_mdl_NI/CAN_Signal/GWM/Other_GWMTx/APIM_Request_Signals_1_FD1 ==
  in : Inport
  ChrgOvrdExitScrn_D_Rq : Subsystem
  EmPrflButtnAssoc_D_Rq : Subsystem
  EmPrflKeyAssoc_D_Rq : Subsystem
  EmPrflNo_D_Rq : Subsystem
  Em_D_Stat : Subsystem
  Rba_D_Rq : Subsystem
  bus_creator : BusCreator  Inputs=6
  bus_selector : BusSelector  OutputSignals=ChrgOvrdExitScrn_D_Rq,EmPrflButtnAssoc_D_Rq,EmPrflKeyAssoc_D_Rq,EmPrflNo_D_Rq,Em_D_Stat,Rba_D_Rq
  out_port : Outport
  wires:
  bus_creator/1 -> out_port/1  "APIM_Request_Signals_1_FD1"
  ChrgOvrdExitScrn_D_Rq/1(out) -> bus_creator/1  "ChrgOvrdExitScrn_D_Rq"
  EmPrflButtnAssoc_D_Rq/1(out) -> bus_creator/2  "EmPrflButtnAssoc_D_Rq"
  EmPrflKeyAssoc_D_Rq/1(out) -> bus_creator/3  "EmPrflKeyAssoc_D_Rq"
  EmPrflNo_D_Rq/1(out) -> bus_creator/4  "EmPrflNo_D_Rq"
  Em_D_Stat/1(out) -> bus_creator/5  "Em_D_Stat"
  Rba_D_Rq/1(out) -> bus_creator/6  "Rba_D_Rq"
  bus_selector/1 -> ChrgOvrdExitScrn_D_Rq/1(in)  "<ChrgOvrdExitScrn_D_Rq>"
  bus_selector/2 -> EmPrflButtnAssoc_D_Rq/1(in)  "<EmPrflButtnAssoc_D_Rq>"
  bus_selector/3 -> EmPrflKeyAssoc_D_Rq/1(in)  "<EmPrflKeyAssoc_D_Rq>"
  bus_selector/4 -> EmPrflNo_D_Rq/1(in)  "<EmPrflNo_D_Rq>"
  bus_selector/5 -> Em_D_Stat/1(in)  "<Em_D_Stat>"
  bus_selector/6 -> Rba_D_Rq/1(in)  "<Rba_D_Rq>"
  in/1 -> bus_selector/1

== system test_mdl_NI/CAN_Signal/GWM/Other_GWMTx/APIM_Request_Signals_FD1 ==
  in : Inport
  CbnCmrtPrefListIndx_Rq : Subsystem
  CbnCmrtPrefLstNmItm_Rq : Subsystem
  ChargePortPwr_Rq : Subsystem
  ChrgStatDsply_D_Rq : Subsystem
  FactoryReset_Rq : Subsystem
  LongTermParking_Rq : Subsystem
  ModemReset_D_Rq : Subsystem
  NextUsageTimeToggle_Rq : Subsystem
  OffPeakTimeSetHR_Rq : Subsystem
  OffPeakTimeSetMin_Rq : Subsystem
  StopStrtDrvMde_B_RqBtn3 : Subsystem
  TCU_ESN_D_Rq : Subsystem
  bus_creator : BusCreator  Inputs=12
  bus_selector : BusSelector  OutputSignals=CbnCmrtPrefListIndx_Rq,CbnCmrtPrefLstNmItm_Rq,ChargePortPwr_Rq,ChrgStatDsply_D_Rq,FactoryReset_Rq,LongTermParking_Rq,ModemReset_D_Rq,NextUsageTimeToggle_Rq,OffPeakTimeSetHR_Rq,OffPeakTimeSetMin_Rq,StopStrtDrvMde_B_RqBtn3,TCU_ESN_D_Rq
  out_port : Outport
  wires:
  bus_creator/1 -> out_port/1  "APIM_Request_Signals_FD1"
  CbnCmrtPrefListIndx_Rq/1(out) -> bus_creator/1  "CbnCmrtPrefListIndx_Rq"
  CbnCmrtPrefLstNmItm_Rq/1(out) -> bus_creator/2  "CbnCmrtPrefLstNmItm_Rq"
  ChargePortPwr_Rq/1(out) -> bus_creator/3  "ChargePortPwr_Rq"
  ChrgStatDsply_D_Rq/1(out) -> bus_creator/4  "ChrgStatDsply_D_Rq"
  FactoryReset_Rq/1(out) -> bus_creator/5  "FactoryReset_Rq"
  LongTermParking_Rq/1(out) -> bus_creator/6  "LongTermParking_Rq"
  ModemReset_D_Rq/1(out) -> bus_creator/7  "ModemReset_D_Rq"
  NextUsageTimeToggle_Rq/1(out) -> bus_creator/8  "NextUsageTimeToggle_Rq"
  OffPeakTimeSetHR_Rq/1(out) -> bus_creator/9  "OffPeakTimeSetHR_Rq"
  OffPeakTimeSetMin_Rq/1(out) -> bus_creator/10  "OffPeakTimeSetMin_Rq"
  StopStrtDrvMde_B_RqBtn3/1(out) -> bus_creator/11  "StopStrtDrvMde_B_RqBtn3"
  TCU_ESN_D_Rq/1(out) -> bus_creator/12  "TCU_ESN_D_Rq"
  bus_selector/1 -> CbnCmrtPrefListIndx_Rq/1(in)  "<CbnCmrtPrefListIndx_Rq>"
  bus_selector/2 -> CbnCmrtPrefLstNmItm_Rq/1(in)  "<CbnCmrtPrefLstNmItm_Rq>"
  bus_selector/3 -> ChargePortPwr_Rq/1(in)  "<ChargePortPwr_Rq>"
  bus_selector/4 -> ChrgStatDsply_D_Rq/1(in)  "<ChrgStatDsply_D_Rq>"
  bus_selector/5 -> FactoryReset_Rq/1(in)  "<FactoryReset_Rq>"
  bus_selector/6 -> LongTermParking_Rq/1(in)  "<LongTermParking_Rq>"
  bus_selector/7 -> ModemReset_D_Rq/1(in)  "<ModemReset_D_Rq>"
  bus_selector/8 -> NextUsageTimeToggle_Rq/1(in)  "<NextUsageTimeToggle_Rq>"
  bus_selector/9 -> OffPeakTimeSetHR_Rq/1(in)  "<OffPeakTimeSetHR_Rq>"
  bus_selector/10 -> OffPeakTimeSetMin_Rq/1(in)  "<OffPeakTimeSetMin_Rq>"
  bus_selector/11 -> StopStrtDrvMde_B_RqBtn3/1(in)  "<StopStrtDrvMde_B_RqBtn3>"
  bus_selector/12 -> TCU_ESN_D_Rq/1(in)  "<TCU_ESN_D_Rq>"
  in/1 -> bus_selector/1

== system test_mdl_NI/CAN_Signal/GWM/Other_GWMTx/APIM_Send_Signals1_FD1 ==
  in : Inport
  APIM_ActiveTrackNum_St : Subsystem
  APIM_NumberofTracks_St : Subsystem
  AutoHoldSwtch_D_Stat3 : Subsystem
  CenterStackRing_D_Actl : Subsystem
  ChrgCordUnlock_B_Rq : Subsystem
  TrlrAidCancl_B_Rq : Subsystem
  TrlrAidSetup_D_Stat : Subsystem
  TrlrTrgtAcquire_D_Rq : Subsystem
  ValetMode_D_Stat : Subsystem
  bus_creator : BusCreator  Inputs=9
  bus_selector : BusSelector  OutputSignals=APIM_ActiveTrackNum_St,APIM_NumberofTracks_St,AutoHoldSwtch_D_Stat3,CenterStackRing_D_Actl,ChrgCordUnlock_B_Rq,TrlrAidCancl_B_Rq,TrlrAidSetup_D_Stat,TrlrTrgtAcquire_D_Rq,ValetMode_D_Stat
  out_port : Outport
  wires:
  bus_creator/1 -> out_port/1  "APIM_Send_Signals1_FD1"
  APIM_ActiveTrackNum_St/1(out) -> bus_creator/1  "APIM_ActiveTrackNum_St"
  APIM_NumberofTracks_St/1(out) -> bus_creator/2  "APIM_NumberofTracks_St"
  AutoHoldSwtch_D_Stat3/1(out) -> bus_creator/3  "AutoHoldSwtch_D_Stat3"
  CenterStackRing_D_Actl/1(out) -> bus_creator/4  "CenterStackRing_D_Actl"
  ChrgCordUnlock_B_Rq/1(out) -> bus_creator/5  "ChrgCordUnlock_B_Rq"
  TrlrAidCancl_B_Rq/1(out) -> bus_creator/6  "TrlrAidCancl_B_Rq"
  TrlrAidSetup_D_Stat/1(out) -> bus_creator/7  "TrlrAidSetup_D_Stat"
  TrlrTrgtAcquire_D_Rq/1(out) -> bus_creator/8  "TrlrTrgtAcquire_D_Rq"
  ValetMode_D_Stat/1(out) -> bus_creator/9  "ValetMode_D_Stat"
  bus_selector/1 -> APIM_ActiveTrackNum_St/1(in)  "<APIM_ActiveTrackNum_St>"
  bus_selector/2 -> APIM_NumberofTracks_St/1(in)  "<APIM_NumberofTracks_St>"
  bus_selector/3 -> AutoHoldSwtch_D_Stat3/1(in)  "<AutoHoldSwtch_D_Stat3>"
  bus_selector/4 -> CenterStackRing_D_Actl/1(in)  "<CenterStackRing_D_Actl>"
  bus_selector/5 -> ChrgCordUnlock_B_Rq/1(in)  "<ChrgCordUnlock_B_Rq>"
  bus_selector/6 -> TrlrAidCancl_B_Rq/1(in)  "<TrlrAidCancl_B_Rq>"
  bus_selector/7 -> TrlrAidSetup_D_Stat/1(in)  "<TrlrAidSetup_D_Stat>"
  bus_selector/8 -> TrlrTrgtAcquire_D_Rq/1(in)  "<TrlrTrgtAcquire_D_Rq>"
  bus_selector/9 -> ValetMode_D_Stat/1(in)  "<ValetMode_D_Stat>"
  in/1 -> bus_selector/1

== system test_mdl_NI/CAN_Signal/GWM/Other_GWMTx/APIM_Send_Signals_2_FD1 ==
  in : Inport
  OnbChrgClearAll_B_Rq : Subsystem
  OnbChrgGoTDelete_B_Rq : Subsystem
  OnbChrgGoTElement_D_Rq : Subsystem
  OnbChrgGoTExtHtr_D_Rq : Subsystem
  OnbChrgGoTHr_T_Rq : Subsystem
  OnbChrgGoTMnte_D_Rq : Subsystem
  OnbChrgGoTOn_D_Rq : Subsystem
  OnbChrgGoTPrcond_D_Rq : Subsystem
  OnbChrgGoTTouch_D_Rq : Subsystem
  OnbChrgGoTUpdate_B_Rq : Subsystem
  OtaTrg_D_Stat : Subsystem
  PaakMyKey_D_Rq : Subsystem
  TCU_Final_Actvtn_St : Subsystem
  TCU_Init_Actvtn_St : Subsystem
  TrlrAidMde_D_Rq : Subsystem
  bus_creator : BusCreator  Inputs=15
  bus_selector : BusSelector  OutputSignals=OnbChrgClearAll_B_Rq,OnbChrgGoTDelete_B_Rq,OnbChrgGoTElement_D_Rq,OnbChrgGoTExtHtr_D_Rq,OnbChrgGoTHr_T_Rq,OnbChrgGoTMnte_D_Rq,OnbChrgGoTOn_D_Rq,OnbChrgGoTPrcond_D_Rq,OnbChrgGoTTouch_D_Rq,OnbChrgGoTUpdate_B_Rq,OtaTrg_D_Stat,PaakMyKey_D_Rq,TCU_Final_Actvtn_St,TCU_Init_Actvtn_St,TrlrAidMde_D_Rq
  out_port : Outport
  wires:
  bus_creator/1 -> out_port/1  "APIM_Send_Signals_2_FD1"
  OnbChrgClearAll_B_Rq/1(out) -> bus_creator/1  "OnbChrgClearAll_B_Rq"
  OnbChrgGoTDelete_B_Rq/1(out) -> bus_creator/2  "OnbChrgGoTDelete_B_Rq"
  OnbChrgGoTElement_D_Rq/1(out) -> bus_creator/3  "OnbChrgGoTElement_D_Rq"
  OnbChrgGoTExtHtr_D_Rq/1(out) -> bus_creator/4  "OnbChrgGoTExtHtr_D_Rq"
  OnbChrgGoTHr_T_Rq/1(out) -> bus_creator/5  "OnbChrgGoTHr_T_Rq"
  OnbChrgGoTMnte_D_Rq/1(out) -> bus_creator/6  "OnbChrgGoTMnte_D_Rq"
  OnbChrgGoTOn_D_Rq/1(out) -> bus_creator/7  "OnbChrgGoTOn_D_Rq"
  OnbChrgGoTPrcond_D_Rq/1(out) -> bus_creator/8  "OnbChrgGoTPrcond_D_Rq"
  OnbChrgGoTTouch_D_Rq/1(out) -> bus_creator/9  "OnbChrgGoTTouch_D_Rq"
  OnbChrgGoTUpdate_B_Rq/1(out) -> bus_creator/10  "OnbChrgGoTUpdate_B_Rq"
  OtaTrg_D_Stat/1(out) -> bus_creator/11  "OtaTrg_D_Stat"
  PaakMyKey_D_Rq/1(out) -> bus_creator/12  "PaakMyKey_D_Rq"
  TCU_Final_Actvtn_St/1(out) -> bus_creator/13  "TCU_Final_Actvtn_St"
  TCU_Init_Actvtn_St/1(out) -> bus_creator/14  "TCU_Init_Actvtn_St"
  TrlrAidMde_D_Rq/1(out) -> bus_creator/15  "TrlrAidMde_D_Rq"
  bus_selector/1 -> OnbChrgClearAll_B_Rq/1(in)  "<OnbChrgClearAll_B_Rq>"
  bus_selector/2 -> OnbChrgGoTDelete_B_Rq/1(in)  "<OnbChrgGoTDelete_B_Rq>"
  bus_selector/3 -> OnbChrgGoTElement_D_Rq/1(in)  "<OnbChrgGoTElement_D_Rq>"
  bus_selector/4 -> OnbChrgGoTExtHtr_D_Rq/1(in)  "<OnbChrgGoTExtHtr_D_Rq>"
  bus_selector/5 -> OnbChrgGoTHr_T_Rq/1(in)  "<OnbChrgGoTHr_T_Rq>"
  bus_selector/6 -> OnbChrgGoTMnte_D_Rq/1(in)  "<OnbChrgGoTMnte_D_Rq>"
  bus_selector/7 -> OnbChrgGoTOn_D_Rq/1(in)  "<OnbChrgGoTOn_D_Rq>"
  bus_selector/8 -> OnbChrgGoTPrcond_D_Rq/1(in)  "<OnbChrgGoTPrcond_D_Rq>"
  bus_selector/9 -> OnbChrgGoTTouch_D_Rq/1(in)  "<OnbChrgGoTTouch_D_Rq>"
  bus_selector/10 -> OnbChrgGoTUpdate_B_Rq/1(in)  "<OnbChrgGoTUpdate_B_Rq>"
  bus_selector/11 -> OtaTrg_D_Stat/1(in)  "<OtaTrg_D_Stat>"
  bus_selector/12 -> PaakMyKey_D_Rq/1(in)  "<PaakMyKey_D_Rq>"
  bus_selector/13 -> TCU_Final_Actvtn_St/1(in)  "<TCU_Final_Actvtn_St>"
  bus_selector/14 -> TCU_Init_Actvtn_St/1(in)  "<TCU_Init_Actvtn_St>"
  bus_selector/15 -> TrlrAidMde_D_Rq/1(in)  "<TrlrAidMde_D_Rq>"
  in/1 -> bus_selector/1

== system test_mdl_NI/CAN_Signal/GWM/Other_GWMTx/ActiveFrontStrg_Stat2_FD1 ==
  in : Inport
  SteWhlRelCalib_An_Sns : Subsystem
  SteWhlRelCalib_T_Actl : Subsystem
  bus_creator : BusCreator  Inputs=2
  bus_selector : BusSelector  OutputSignals=SteWhlRelCalib_An_Sns,SteWhlRelCalib_T_Actl
  out_port : Outport
  wires:
  bus_creator/1 -> out_port/1  "ActiveFrontStrg_Stat2_FD1"
  SteWhlRelCalib_An_Sns/1(out) -> bus_creator/1  "SteWhlRelCalib_An_Sns"
  SteWhlRelCalib_T_Actl/1(out) -> bus_creator/2  "SteWhlRelCalib_T_Actl"
  bus_selector/1 -> SteWhlRelCalib_An_Sns/1(in)  "<SteWhlRelCalib_An_Sns>"
  bus_selector/2 -> SteWhlRelCalib_T_Actl/1(in)  "<SteWhlRelCalib_T_Actl>"
  in/1 -> bus_selector/1

== system test_mdl_NI/CAN_Signal/GWM/Other_GWMTx/ActiveFrontStrg_Stat_FD1 ==
  in : Inport
  SteWhlBrkAnActl_No_Cnt : Subsystem
  SteWhlBrkAnActl_No_Cs : Subsystem
  SteWhlBrkOffst_An_Actl : Subsystem
  SteWhlOffstRq_D_Stat : Subsystem
  SteWhlOffst_An_TotActl : Subsystem
  bus_creator : BusCreator  Inputs=5
  bus_selector : BusSelector  OutputSignals=SteWhlBrkAnActl_No_Cnt,SteWhlBrkAnActl_No_Cs,SteWhlBrkOffst_An_Actl,SteWhlOffstRq_D_Stat,SteWhlOffst_An_TotActl
  out_port : Outport
  wires:
  bus_creator/1 -> out_port/1  "ActiveFrontStrg_Stat_FD1"
  SteWhlBrkAnActl_No_Cnt/1(out) -> bus_creator/1  "SteWhlBrkAnActl_No_Cnt"
  SteWhlBrkAnActl_No_Cs/1(out) -> bus_creator/2  "SteWhlBrkAnActl_No_Cs"
  SteWhlBrkOffst_An_Actl/1(out) -> bus_creator/3  "SteWhlBrkOffst_An_Actl"
  SteWhlOffstRq_D_Stat/1(out) -> bus_creator/4  "SteWhlOffstRq_D_Stat"
  SteWhlOffst_An_TotActl/1(out) -> bus_creator/5  "SteWhlOffst_An_TotActl"
  bus_selector/1 -> SteWhlBrkAnActl_No_Cnt/1(in)  "<SteWhlBrkAnActl_No_Cnt>"
  bus_selector/2 -> SteWhlBrkAnActl_No_Cs/1(in)  "<SteWhlBrkAnActl_No_Cs>"
  bus_selector/3 -> SteWhlBrkOffst_An_Actl/1(in)  "<SteWhlBrkOffst_An_Actl>"
  bus_selector/4 -> SteWhlOffstRq_D_Stat/1(in)  "<SteWhlOffstRq_D_Stat>"
  bus_selector/5 -> SteWhlOffst_An_TotActl/1(in)  "<SteWhlOffst_An_TotActl>"
  in/1 -> bus_selector/1

== system test_mdl_NI/CAN_Signal/GWM/Other_GWMTx/AllTerrainControlData_FD1 ==
  in : Inport
  SelDrvMdeCnt_D_Stat : Subsystem
  SelDrvMdeSwtchOk_D_Stat : Subsystem
  SelDrvMdeSwtch_D_Stat : Subsystem
  SelDrvMdeSwtch_No_Actl : Subsystem
  bus_creator : BusCreator  Inputs=4
  bus_selector : BusSelector  OutputSignals=SelDrvMdeCnt_D_Stat,SelDrvMdeSwtchOk_D_Stat,SelDrvMdeSwtch_D_Stat,SelDrvMdeSwtch_No_Actl
  out_port : Outport
  wires:
  bus_creator/1 -> out_port/1  "AllTerrainControlData_FD1"
  SelDrvMdeCnt_D_Stat/1(out) -> bus_creator/1  "SelDrvMdeCnt_D_Stat"
  SelDrvMdeSwtchOk_D_Stat/1(out) -> bus_creator/2  "SelDrvMdeSwtchOk_D_Stat"
  SelDrvMdeSwtch_D_Stat/1(out) -> bus_creator/3  "SelDrvMdeSwtch_D_Stat"
  SelDrvMdeSwtch_No_Actl/1(out) -> bus_creator/4  "SelDrvMdeSwtch_No_Actl"
  bus_selector/1 -> SelDrvMdeCnt_D_Stat/1(in)  "<SelDrvMdeCnt_D_Stat>"
  bus_selector/2 -> SelDrvMdeSwtchOk_D_Stat/1(in)  "<SelDrvMdeSwtchOk_D_Stat>"
  bus_selector/3 -> SelDrvMdeSwtch_D_Stat/1(in)  "<SelDrvMdeSwtch_D_Stat>"
  bus_selector/4 -> SelDrvMdeSwtch_No_Actl/1(in)  "<SelDrvMdeSwtch_No_Actl>"
  in/1 -> bus_selector/1

== system test_mdl_NI/CAN_Signal/GWM/Other_GWMTx/All_Terrain_Data_FD1 ==
  in : Inport
  TerrMde_D_RqDrv : Subsystem
  TerrStat_D_RqDsply : Subsystem
  bus_creator : BusCreator  Inputs=2
  bus_selector : BusSelector  OutputSignals=TerrMde_D_RqDrv,TerrStat_D_RqDsply
  out_port : Outport
  wires:
  bus_creator/1 -> out_port/1  "All_Terrain_Data_FD1"
  TerrMde_D_RqDrv/1(out) -> bus_creator/1  "TerrMde_D_RqDrv"
  TerrStat_D_RqDsply/1(out) -> bus_creator/2  "TerrStat_D_RqDsply"
  bus_selector/1 -> TerrMde_D_RqDrv/1(in)  "<TerrMde_D_RqDrv>"
  bus_selector/2 -> TerrStat_D_RqDsply/1(in)  "<TerrStat_D_RqDsply>"
  in/1 -> bus_selector/1
